simulink model "power_currmeasure"  (Simulink 6.0)
settings: Solver=ode23s  SolverMode=SingleTasking  StartTime=0.0  StopTime=0.1  RelTol=1e-3  AbsTol=1e-6
libraries: powerlib x14
settings Model: Creator=patrice  LastModifiedBy=batserve  ExtModeTrigMode=oneshot  ExtModeArmWhenConnect=off  ExtModeAutoUpdateStatusClock=off
settings DataIOCC: LimitDataPoints=off  SignalLoggingName=sigsOut
settings OptimizationCC: BooleanDataType=off
settings DebuggingCC: SolverPrmCheckMsg=none
settings HardwareCC: TargetUnknown=on
settings RTWCC: TemplateMakefile=grt_unix.tmf

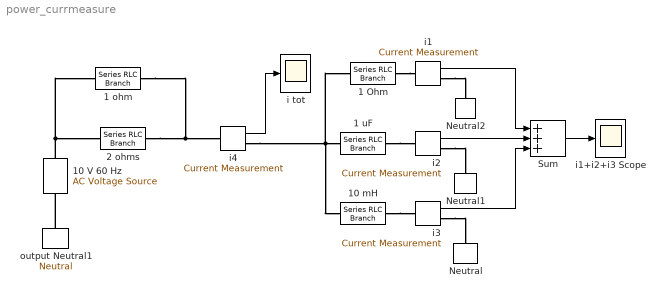
== system power_currmeasure ==
  1 Ohm : powerlib/Elements/Series RLC Branch  PhysicalDomain=powersysdomain  SubClassName=unknown  PortType=p1  LConnTagsString=__new0  RConnTagsString=__new0  Resistance=1  Inductance=0  Capacitance=inf  Measurements=None
  1 ohm : powerlib/Elements/Series RLC Branch  PhysicalDomain=powersysdomain  SubClassName=unknown  PortType=p1  LConnTagsString=__new0  RConnTagsString=__new0  Resistance=1  Inductance=0  Capacitance=inf  Measurements=None
  1 uF : powerlib/Elements/Series RLC Branch  PhysicalDomain=powersysdomain  SubClassName=unknown  PortType=p1  LConnTagsString=__new0  RConnTagsString=__new0  Resistance=0  Inductance=0  Capacitance=1e-6  Measurements=None
  10 V 60 Hz : powerlib/Electrical Sources/AC Voltage Source  Description=source block  Orientation=up  Amplitude=10  Phase=0  Frequency=60  SampleTime=0  Measurements=None
      settings: AttributesFormatString=\n
  10 mH : powerlib/Elements/Series RLC Branch  PhysicalDomain=powersysdomain  SubClassName=unknown  PortType=p1  LConnTagsString=__new0  RConnTagsString=__new0  Resistance=0  Inductance=10  Capacitance=inf  Measurements=None
  2 ohms : powerlib/Elements/Series RLC Branch  PhysicalDomain=powersysdomain  SubClassName=unknown  PortType=p1  LConnTagsString=__new0  RConnTagsString=__new0  Resistance=2  Inductance=0  Capacitance=inf  Measurements=None
  Neutral : powerlib/Elements/Neutral  Orientation=down  PhysicalDomain=powersysdomain  SubClassName=unknown  PortType=p1  LConnTagsString=a  NodeNumber=50
  Neutral1 : powerlib/Elements/Neutral  Orientation=down  PhysicalDomain=powersysdomain  SubClassName=unknown  PortType=p1  LConnTagsString=a  NodeNumber=50
  Neutral2 : powerlib/Elements/Neutral  Orientation=down  PhysicalDomain=powersysdomain  SubClassName=unknown  PortType=p1  LConnTagsString=a  NodeNumber=50
  Sum : Sum  Inputs=+++  SaturateOnIntegerOverflow=on  InputSameDT=on
  i tot : Scope
      settings: TickLabels=on  TimeRange=0.1  YMin=-12  YMax=12  DataFormat=Array
  i{1..4} (4 alike) : powerlib/Measurements/Current Measurement  Tag=PoWeRsYsTeMmEaSuReMeNt  PhasorSimulation=off  OutputType=Magnitude  PSBequivalent=0
  i1+i2+i3 Scope : Scope
      settings: TickLabels=on  TimeRange=0.1  YMin=-12  YMax=12  DataFormat=Array
  output Neutral1 : powerlib/Elements/Neutral  Orientation=down  PhysicalDomain=powersysdomain  SubClassName=unknown  PortType=p1  LConnTagsString=a  NodeNumber=50
  wires:
  Sum/1 -> i1+i2+i3 Scope/1
  i4/1 -> i tot/1
  i3/1 -> Sum/3
  i2/1 -> Sum/2
  i1/1 -> Sum/1
  connections:
  10 V 60 Hz/RConn1 -- 1 ohm/LConn1 -- 2 ohms/LConn1
  output Neutral1/LConn1 -- 10 V 60 Hz/LConn1
  2 ohms/RConn1 -- i4/LConn1 -- 1 ohm/RConn1
  1 uF/LConn1 -- 1 Ohm/LConn1 -- 10 mH/LConn1 -- i4/RConn1
  i3/RConn1 -- Neutral/LConn1
  i2/RConn1 -- Neutral1/LConn1
  i1/RConn1 -- Neutral2/LConn1
  1 uF/RConn1 -- i2/LConn1
  1 Ohm/RConn1 -- i1/LConn1
  10 mH/RConn1 -- i3/LConn1
